simulink model "IntegratedStarterGenerator_lithium_ion"  (R2024b)
settings: Solver=ode23tb  StartTime=0.0  StopTime=15  FixedStep=1e-6  RelTol=1e-4  EnableMultiTasking=on
PreLoadFcn:
  | BeltStarterGeneratorData;
model workspace (MAT data in the model file):
  Cdc = 0.001
  ID_MAP = [-155.095933536 -155.095933536 -155.095933536 -155.095933536 -155.095933536 -155.095933536 -155.095933536 -155.095933536 -200.847752045 -245.560073478 -288.511134519 -330.698372533 ... (48076 elements, 28x101x17)]
  IQ_MAP = [-234.678365656 -234.678365656 -234.678365656 -234.678365656 -234.678365656 -234.678365656 -234.678365656 -234.678365656 -207.892729616 -187.030522468 -170.586354015 -157.025794022 ... (48076 elements, 28x101x17)]
  Ki_dcdc = 10
  Ki_id = 170
  Ki_iq = 170
  Ki_vdc = 100
  Kp_dcdc = 0.5
  Kp_id = 0.24
  Kp_iq = 0.24
  Kp_vdc = 20
  L0 = 5e-05
  Ld = 0.00011
  Lq = 0.00011
  Pmax = 140
  RPM_VECT = [0 1000 2000 3000 4000 5000 6000 7000 8000 9000 10000]
  R_f : Simulink.Parameter (value not decoded)
  Rs = 0.085
  TQ_VECT = [-3.5 -3.43 -3.36 -3.29 -3.22 -3.15 -3.08 -3.01 -2.94 -2.87 -2.8 -2.73 ... (101 elements, 1x101)]
  Tmax = 3.5
  Ts = 5e-06
  Tsi = 0.0001
  VDC_VECT = [8 8.625 9.25 9.875 10.5 11.125 11.75 12.375 13 13.625 14.25 14.875 ... (17 elements, 1x17)]
  dend_id = [1 -0.966796355036]
  dend_iq = [1 -0.900395111642]
  fsw = 5000
  fswd = 5000
  numd_id = 0.0332036449638
  numd_iq = 0.099604888358
  p = 3
  psim = 0.0159
  r_tire : Simulink.Parameter (value not decoded)
  tout = [0 5e-06 1e-05 1.5e-05 2e-05 2.5e-05 3e-05 3.5e-05 4e-05 4.5e-05 5e-05 5.5e-05 ... (200005 elements, 200005x1)]
symbols that are objects in the model workspace (value not decoded): R_f, r_tire
undefined symbols (not defined in the file or in its folder): DiscIntNeverNeededParam
libraries: fl_lib x51, nesl_utility x26, simulink x12, ee_lib x6, eeDiscretePi x3, sdl_lib x2, eeTransforms x2, batteryecm_lib x1, eePmsmCurrentController x1, eePmsmCurrentReferenceGen x1, eePmsmTorqueEstimator x1, eePwmGeneratorTwoLevel x1
(part 2 of 3)

== system IntegratedStarterGenerator_lithium_ion/Current sensor ==
  Current Sensor : fl_lib/Electrical/Electrical Sensors/Current Sensor
  PS-Simulink Converter1 : nesl_utility/PS-Simulink Converter  PhysicalDomain=network_engine_domain  SubClassName=ps_output  LeftPortType=input  RightPortType=output  PseudoPeriodic=off  Frequencies=[]  VectorFormat=1-D array  Unit=A  AffineConversion=off
  + : PMIOPort  Side=Left
  - : PMIOPort  Port=2  Side=Right
  tag scope: i_batt=global
  wires:
  PS-Simulink Converter1/1 -> [i_batt]
  connections:
  Current Sensor/RConn1 -- PS-Simulink Converter1/LConn1
  Current Sensor/LConn1 -- +/RConn1
  -/RConn1 -- Current Sensor/RConn2

== system IntegratedStarterGenerator_lithium_ion/Current sensor1 ==
  Current Sensor : fl_lib/Electrical/Electrical Sensors/Current Sensor
  PS-Simulink Converter1 : nesl_utility/PS-Simulink Converter  PhysicalDomain=network_engine_domain  SubClassName=ps_output  LeftPortType=input  RightPortType=output  PseudoPeriodic=off  Frequencies=[]  VectorFormat=1-D array  Unit=A  AffineConversion=off
  + : PMIOPort  Side=Left
  - : PMIOPort  Port=2  Side=Right
  tag scope: idc=global
  wires:
  PS-Simulink Converter1/1 -> [idc]
  connections:
  Current Sensor/RConn1 -- PS-Simulink Converter1/LConn1
  Current Sensor/LConn1 -- +/RConn1
  -/RConn1 -- Current Sensor/RConn2

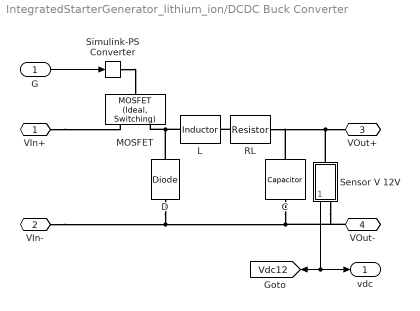
== system IntegratedStarterGenerator_lithium_ion/DCDC Buck Converter ==
  G : Inport
  C : fl_lib/Electrical/Electrical Elements/Capacitor  c=100 uF  r=1e-6 Ohm  g=0 1/Ohm  i_specify=off  i_priority=None  i=0 A  i_nominal_specify=off  i_nominal_value=1  i_nominal_unit=A  v_specify=off  v_priority=None  v=0 V  v_nominal_specify=off  v_nominal_value=1  v_nominal_unit=V  vc_specify=on  vc_priority=Low  vc=0 V  vc_nominal_specify=off  vc_nominal_value=1  vc_nominal_unit=V
  D : fl_lib/Electrical/Electrical Elements/Diode  Vf=0.6 V  Ron=0.3 Ohm  Goff=1e-8 1/Ohm  i_specify=off  i_priority=None  i=0 A  i_nominal_specify=off  i_nominal_value=1  i_nominal_unit=A  v_specify=off  v_priority=None  v=0 V  v_nominal_specify=off  v_nominal_value=1  v_nominal_unit=V
  L : fl_lib/Electrical/Electrical Elements/Inductor  l=3.7 mH  r=0 Ohm  g=1e-9 1/Ohm  i_specify=off  i_priority=None  i=0 A  i_nominal_specify=off  i_nominal_value=1  i_nominal_unit=A  v_specify=off  v_priority=None  v=0 V  v_nominal_specify=off  v_nominal_value=1  v_nominal_unit=V  i_L_specify=on  i_L_priority=Low  i_L=0 A  i_L_nominal_specify=off  i_L_nominal_value=1  i_L_nominal_unit=A
  MOSFET : ee_lib/Semiconductors & Converters/MOSFET (Ideal, Switching)  port_option=ee.enum.controlport.ps  Rds=0.01 Ohm  Goff=1e-6 1/Ohm  Vth=0.5 V  diode_param=2  diode_Vf=0.8 V  diode_Ron=0.001 Ohm  diode_Goff=1e-5 1/Ohm  diode_C=5e-8 F  diode_iRM=-235 A  diode_iF=300 A  diode_idot=-50 A/us  diode_trr_param=1  diode_trr_factor=3  diode_trr=15 us  diode_Qrr=1.5e+3 s*uA  ids_specify=off  ids_priority=None  ids=0 A  ids_nominal_specify=off  ids_nominal_value=1  ids_nominal_unit=A  vds_specify=off  vds_priority=None  vds=0 V  vds_nominal_specify=off  vds_nominal_value=1  vds_nominal_unit=V  vgs_specify=off  vgs_priority=None  vgs=0 V  vgs_nominal_specify=off  vgs_nominal_value=1  vgs_nominal_unit=V  thermal_loss_option=ee.enum.converters.thermalLossOption.constantvalues  Von_data=[0, 1.1, 1.3, 1.45, 1.75, 2.25, 2.7; 0, 1, 1.15, 1.35, 1.7, 2.35, 3] V  Tj=[298.15, 398.15] K  Iout_data=[0, 10, 50, 100, 200, 400, 600] A  Eon_data=[0, .29, 1.43, 2.86, 5.71, 13.14, 22.86; 0, .57, 2.63, 5.14, 10.29, 20.57, 30.29] * 1e-3 J  Eoff_data=[0, .21, 1.07, 2.14, 4.29, 9.86, 17.14; 0, .43, 1.97, 3.86, 7.71, 15.43, 22.71] * 1e-3 J  Eon_data_3D=[zeros(2, 5, 3)] J  Eoff_data_3D=[zeros(2, 5, 3)] J  Tj_loss=[298.15, 398.15] K  Iout_data_loss=[0, 10, 50, 100, 200, 400, 600] A  tabulateWithVds=false  Vds_loss=[0, 150, 300] V  Eon_scalar=22.86e-3 J  Eoff_scalar=17.14e-3 J  Voff=300 V  Iout_scalar=600 A  useCurrentFromPreviousCycle=false  useVoltageFromPreviousCycle=false  diodeModelType=ee.enum.converters.diodeModelType.pwl  diodeTableType=ee.enum.diode.tableType.IfMat  diode_ReverseIVType=ee.enum.diode.diodeReverseIV.constant  diode_IfMat=[.07, .12, .19, 1.75, 4.24, 7.32, 11.2; .16, .3, .72, 2.14, 4.02, 6.35, 9.12] A  diode_VfMat=[.9, 1.15, 1.25, 1.5, 1.75, 2.17, 2.6, 2.85; .58, .68, .75, 1.1, 1.38, 1.77, 2.27, 2.7] V  diode_TjVec=[25, 125] degC  diode_VfVec=[.5, .7, .9, 1.3, 1.7, 2.1, 2.5] V  diode_IfVec=[.1, .2, .5, 1, 2, 4, 7, 10] A  diode_IrMat=[1e-06, 2e-06, 5e-06, 1e-05, 2.5e-05, 5e-05, .0001; 2e-06, 5e-06, 1e-05, 4e-05, 8e-05, .0002, .0005] A  diode_VrMat=[10, 100, 200, 250, 300, 325, 350; 10, 70, 160, 220, 270, 300, 320] V  diode_VrVec=[10, 20, 40, 50, 70, 80, 100] V  diode_IrVec=[1e-06, 2e-06, 5e-06, 1e-05, 2e-05, 5e-05, .0001] A  diode_Vr=-600 V  diode_Ls=150 nH  diode_Erec=0.03 J  diode_rec_loss_model=ee.enum.diode.reverseRecoveryModel.fixed  diode_ErecVal=0 J  diode_scaleWithIandV=true  diode_ErecMat=zeros(2, 3) J  diode_TjrecVec=[298.15, 398.15] K  diode_IfrecVec=[.1, 1, 10] A  diode_IrecVal=10 A  diode_VrecVal=10 V  diode_tFilter=1 / 1000 / 100 s  separateThermalPortForDiode=false  thermal_network_parameterization=ee.enum.thermalNetworkTopology.external  Rth=[.03, .2] K/W  Rth_Cauer=[.03, .1, .2] K/W  Rth_Foster=[.03, .2] K/W  thermal_mass_parameterization=ee.enum.thermalNetwork.timeconstant  thermal_mass=[3, 25] J/K  thermal_mass_Cauer=[3, 10, 25] J/K  thermal_mass_Foster=[33, 50] J/K  thermal_time_constant=[.1, 5] s  thermal_time_constant_Cauer=[.1, 1, 5] s  thermal_time_constant_Foster=[1, 10] s  thermal_mass_initial_temperatures=[25, 25] degC  thermal_mass_initial_temperatures_Cauer=[25, 25, 25] degC  junction_thermal_mass=0.1 J/K  Tvec_initial_Foster=[25, 25, 25, 25] degC  RthDiode=[.03, .2] K/W  RthCauerDiode=[.03, .1, .2] K/W  RthFosterDiode=[.03, .2] K/W  thermalMassDiode=[3, 25] J/K  thermalMassCauerDiode=[3, 10, 25] J/K  thermalMassFosterDiode=[33, 50] J/K  thermalTauDiode=[.1, 5] s  thermalTauCauerDiode=[.1, 1, 5] s  thermalTauFosterDiode=[1, 10] s  thermalMassInitTempDiode=[25, 25] degC  thermalMassInitTempCauerDiode=[25, 25, 25] degC  junctionthermalMassDiode=0.1 J/K  TVecInitialFosterDiode=[25, 25, 25, 25] degC  no_thermal_network=0  mosfet_junction_temperature_specify=off  mosfet_junction_temperature_priority=None  mosfet_junction_temperature=25 degC  mosfet_junction_temperature_nominal_specify=off  mosfet_junction_temperature_nominal_value=1  mosfet_junction_temperature_nominal_unit=degC  diode_junction_temperature_specify=off  diode_junction_temperature_priority=None  diode_junction_temperature=25 degC  diode_junction_temperature_nominal_specify=off  diode_junction_temperature_nominal_value=1  diode_junction_temperature_nominal_unit=degC  Qj_specify=off  Qj_priority=None  Qj=0 W  Qj_nominal_specify=off  Qj_nominal_value=1  Qj_nominal_unit=W  accumulatedSwitchingLosses_specify=off  accumulatedSwitchingLosses_priority=None  accumulatedSwitchingLosses=0 J
  RL : fl_lib/Electrical/Electrical Elements/Resistor  R=1.5 Ohm  i_specify=off  i_priority=None  i=0 A  i_nominal_specify=off  i_nominal_value=1  i_nominal_unit=A  v_specify=off  v_priority=None  v=0 V  v_nominal_specify=off  v_nominal_value=1  v_nominal_unit=V
  Sensor V 12V : Subsystem
  Simulink-PS Converter : nesl_utility/Simulink-PS Converter  PhysicalDomain=network_engine_domain  SubClassName=ps_input  LeftPortType=input  RightPortType=output  PseudoPeriodic=off  Frequencies=[]  NoiseDistribution=none  NoiseParameters=[]  Unit=1  AffineConversion=off  FilteringAndDerivatives=zero  SimscapeFilterOrder=1  InputFilterTimeConstant=0.001  UdotUserProvided=1
  VIn+ : PMIOPort  Side=Left
  VIn- : PMIOPort  Port=2  Side=Left
  VOut+ : PMIOPort  Port=3  Side=Right
  VOut- : PMIOPort  Port=4  Side=Right
  vdc : Outport  VectorParamsAs1DForOutWhenUnconnected=off
  tag scope: Vdc12=global
  wires:
  G/1 -> Simulink-PS Converter/1
  Sensor V 12V/1(vdc) -> [Vdc12], vdc/1
  connections:
  VIn-/RConn1 -- D/LConn1 -- Sensor V 12V/RConn1 -- VOut-/RConn1 -- C/RConn1
  Simulink-PS Converter/RConn1 -- MOSFET/LConn1
  L/LConn1 -- D/RConn1 -- MOSFET/RConn2
  VIn+/RConn1 -- MOSFET/RConn1
  RL/LConn1 -- L/RConn1
  C/LConn1 -- RL/RConn1 -- VOut+/RConn1 -- Sensor V 12V/LConn1

== system IntegratedStarterGenerator_lithium_ion/DCDC Controller ==
  Ref : Inport
  Vdc : Inport  Port=2
  Constant : Constant  Value=0  SampleTime=-1
  Discrete PI Controller with Integral Anti-Windup : eeDiscretePi/Discrete PI Controller with Integral Anti-Windup  Kp=Kp_dcdc  Ki=Ki_dcdc  x0=0  B=1  A=0  Ts=1e-3
  PWM Generation : Subsystem  mask{f=fswd, Ts=Ts}
      mask prompts: f "Switching frequency"; Ts "Sample time"
  Rate Transition : RateTransition  OutPortSampleTime=1e-3
  Rate Transition2 : RateTransition
  Sum : Sum  Inputs=|+-
  G : Outport  VectorParamsAs1DForOutWhenUnconnected=off
  wires:
  Vdc/1 -> Rate Transition/1
  Rate Transition2/1 -> PWM Generation/1(DC)
  Ref/1 -> Sum/1
  Rate Transition/1 -> Sum/2
  PWM Generation/1(PWM) -> G/1
  Sum/1 -> Discrete PI Controller with Integral Anti-Windup/1
  Discrete PI Controller with Integral Anti-Windup/1 -> Rate Transition2/1
  Constant/1 -> Discrete PI Controller with Integral Anti-Windup/2

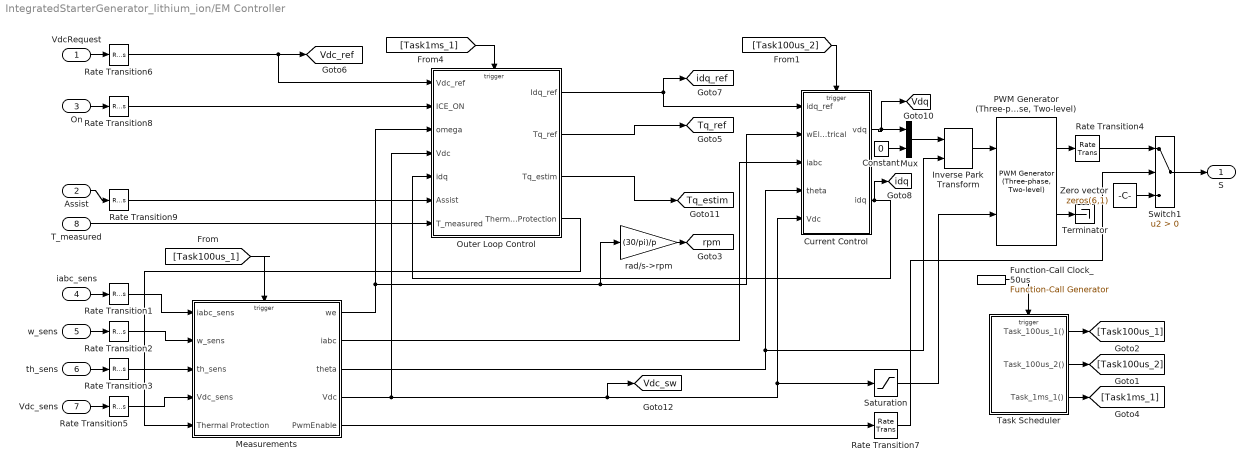
== system IntegratedStarterGenerator_lithium_ion/EM Controller ==
  VdcRequest : Inport
  Assist : Inport  Port=2
  On : Inport  Port=3
  iabc_sens : Inport  Port=4
  w_sens : Inport  Port=5
  th_sens : Inport  Port=6
  Vdc_sens : Inport  Port=7
  T_measured : Inport  Port=8
  Constant : Constant  Value=0  SampleTime=-1
  Current Control : Subsystem
  Function-Call Clock_50us : simulink/Ports & Subsystems/Function-Call Generator  sample_time=5e-5  numberOfIterations=1  DisallowWideOutput=off
  Inverse Park Transform : eeTransforms/Inverse Park Transform  AxisAlignment=Q-axis  PowerInvariant=off
  Measurements : Subsystem
  Mux : Mux  Inputs=2
  Outer Loop Control : Subsystem
  "PWM Generator (Three-phase, Two-level)" : eePwmGeneratorTwoLevel/PWM Generator (Three-phase, Two-level)  PWMMode=Continuous PWM (CPWM)  CPWMMode=SPWM: sinusoidal PWM  DPWMMode=60 DPWM: 60 degree discontinuous PWM  fsw=fsw  Ts=Ts
  Rate Transition{1..9} (9 alike) : RateTransition
  Saturation : Saturate  UpperLimit=500  LowerLimit=10
  Switch1 : Switch  Criteria=u2 > Threshold  SaturateOnIntegerOverflow=off  InputSameDT=off
  Task Scheduler : Stateflow chart  TreatAsAtomicUnit=on
  Terminator : Terminator
  Zero vector : Constant  Value=zeros(6,1)
  rad/s->rpm : Gain  Gain=(30/pi)/p
  S : Outport  VectorParamsAs1DForOutWhenUnconnected=off
  tag scope: Tq_estim=global, Tq_ref=global, Vdc_ref=global, Vdc_sw=global, Vdq=global, idq=global, idq_ref=global, rpm=global
  wires:
  Measurements/4(Vdc) -> Current Control/5(Vdc), Saturation/1, [Vdc_sw], Outer Loop Control/4(Vdc)
  [Task1ms_1] -> Outer Loop Control/Trigger
  Rate Transition8/1 -> Outer Loop Control/2(ICE_ON)
  Rate Transition1/1 -> Measurements/1(iabc_sens)
  Switch1/1 -> S/1
  Rate Transition5/1 -> Measurements/4(Vdc_sens)
  Current Control/1(vdq) -> [Vdq], Mux/1
  Current Control/2(idq) -> [idq], Outer Loop Control/5(idq)
  Outer Loop Control/1(Idq_ref) -> [idq_ref], Current Control/1(idq_ref)
  Task Scheduler/1(Task_100us_1()) -> [Task100us_1]
  Measurements/3(theta) -> Current Control/4(theta), Inverse Park Transform/2
  Rate Transition4/1 -> Switch1/1
  Outer Loop Control/3(Tq_estim) -> [Tq_estim]
  Rate Transition7/1 -> Switch1/2
  VdcRequest/1 -> Rate Transition6/1
  Zero vector/1 -> Switch1/3
  Measurements/1(we) -> Outer Loop Control/3(omega), Current Control/2(wElectrical), rad/s->rpm/1
  th_sens/1 -> Rate Transition3/1
  On/1 -> Rate Transition8/1
  Outer Loop Control/2(Tq_ref) -> [Tq_ref]
  Rate Transition6/1 -> [Vdc_ref], Outer Loop Control/1(Vdc_ref)
  iabc_sens/1 -> Rate Transition1/1
  Task Scheduler/3(Task_1ms_1()) -> [Task1ms_1]
  Rate Transition3/1 -> Measurements/3(th_sens)
  Function-Call Clock_50us/1 -> Task Scheduler/Trigger
  Measurements/5(PwmEnable) -> Rate Transition7/1
  "PWM Generator (Three-phase, Two-level)"/2 -> Terminator/1
  Rate Transition2/1 -> Measurements/2(w_sens)
  Saturation/1 -> "PWM Generator (Three-phase, Two-level)"/2
  [Task100us_2] -> Current Control/Trigger
  w_sens/1 -> Rate Transition2/1
  rad/s->rpm/1 -> [rpm]
  Inverse Park Transform/1 -> "PWM Generator (Three-phase, Two-level)"/1
  "PWM Generator (Three-phase, Two-level)"/1 -> Rate Transition4/1
  Vdc_sens/1 -> Rate Transition5/1
  Task Scheduler/2(Task_100us_2()) -> [Task100us_2]
  [Task100us_1] -> Measurements/Trigger
  Measurements/2(iabc) -> Current Control/3(iabc)
  Mux/1 -> Inverse Park Transform/1
  Constant/1 -> Mux/2
  Assist/1 -> Rate Transition9/1
  Rate Transition9/1 -> Outer Loop Control/6(Assist)
  T_measured/1 -> Outer Loop Control/7(T_measured)
  Outer Loop Control/4(Thermal Protection) -> Measurements/5(Thermal Protection)

== system IntegratedStarterGenerator_lithium_ion/Gate Driver ==
  S : Inport
  Demux : Demux  Outputs=6
  Simulink-PS Converter{1..6} (6 alike) : nesl_utility/Simulink-PS Converter  PhysicalDomain=network_engine_domain  SubClassName=ps_input  LeftPortType=input  RightPortType=output  PseudoPeriodic=off  Frequencies=[]  NoiseDistribution=none  NoiseParameters=[]  Unit=1  AffineConversion=off  FilteringAndDerivatives=zero  SimscapeFilterOrder=1  InputFilterTimeConstant=0.001  UdotUserProvided=1
  Six-Pulse Gate Multiplexer : ee_lib/Semiconductors & Converters/Converters/Six-Pulse Gate Multiplexer  port_option=ee.enum.controlport.ps
  G : PMIOPort  Side=Right
  wires:
  Demux/1 -> Simulink-PS Converter1/1
  S/1 -> Demux/1
  Demux/4 -> Simulink-PS Converter4/1
  Demux/2 -> Simulink-PS Converter2/1
  Demux/3 -> Simulink-PS Converter3/1
  Demux/5 -> Simulink-PS Converter5/1
  Demux/6 -> Simulink-PS Converter6/1
  connections:
  Six-Pulse Gate Multiplexer/RConn1 -- G/RConn1
  Simulink-PS Converter1/RConn1 -- Six-Pulse Gate Multiplexer/LConn1
  Simulink-PS Converter3/RConn1 -- Six-Pulse Gate Multiplexer/LConn3
  Simulink-PS Converter5/RConn1 -- Six-Pulse Gate Multiplexer/LConn5
  Simulink-PS Converter6/RConn1 -- Six-Pulse Gate Multiplexer/LConn6
  Simulink-PS Converter4/RConn1 -- Six-Pulse Gate Multiplexer/LConn4
  Simulink-PS Converter2/RConn1 -- Six-Pulse Gate Multiplexer/LConn2

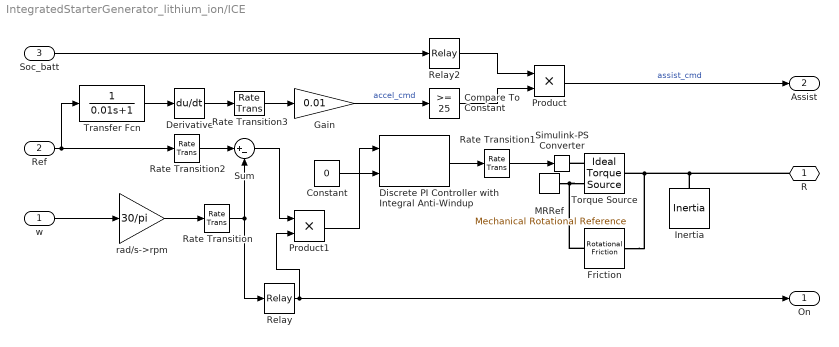
== system IntegratedStarterGenerator_lithium_ion/ICE ==
  w : Inport
  Ref : Inport  Port=2
  Soc_batt : Inport  Port=3
  Compare To Constant : simulink/Logic and Bit Operations/Compare To Constant  relop=>=  const=25  OutDataTypeStr=boolean
  Constant : Constant  Value=0  SampleTime=0.01
  Derivative : Derivative  CoefficientInTFapproximation=0.05
  Discrete PI Controller with Integral Anti-Windup : eeDiscretePi/Discrete PI Controller with Integral Anti-Windup  Kp=0.5  Ki=0.4  x0=0  B=6.5  A=-0.1*Tmax  Ts=0.0001
  Friction : fl_lib/Mechanical/Rotational Elements/Rotational Friction  brkwy_trq=0.01e-3 N*m  brkwy_vel=0.05 rad/s  Col_trq=0.01e-3 N*m  visc_coef=0.0005 N*m/(rad/s)  w_specify=off  w_priority=None  w=0 rad/s  w_nominal_specify=off  w_nominal_value=1  w_nominal_unit=rad/s  t_specify=off  t_priority=None  t=0 N*m  t_nominal_specify=off  t_nominal_value=1  t_nominal_unit=N*m
  Gain : Gain  Gain=0.01
  Inertia : fl_lib/Mechanical/Rotational Elements/Inertia  inertia=0.0025 kg*m^2  num_ports=foundation.enum.numPorts2.one  w_specify=on  w_priority=Low  w=0 rad/s  w_nominal_specify=off  w_nominal_value=1  w_nominal_unit=rad/s  t_specify=off  t_priority=None  t=0 N*m  t_nominal_specify=off  t_nominal_value=1  t_nominal_unit=N*m
  MRRef : fl_lib/Mechanical/Rotational Elements/Mechanical Rotational Reference
  Product : Product
  Product1 : Product
  Rate Transition : RateTransition  OutPortSampleTime=0.0001
  Rate Transition1 : RateTransition
  Rate Transition2 : RateTransition  OutPortSampleTime=0.0001
  Rate Transition3 : RateTransition  OutPortSampleTime=0.0001
  Relay : Relay  OnSwitchValue=950  OffSwitchValue=850  ZeroCross=off
  Relay2 : Relay  OnSwitchValue=0.5  OffSwitchValue=0.2  ZeroCross=off
  Simulink-PS Converter : nesl_utility/Simulink-PS Converter  PhysicalDomain=network_engine_domain  SubClassName=ps_input  LeftPortType=input  RightPortType=output  PseudoPeriodic=off  Frequencies=[]  NoiseDistribution=none  NoiseParameters=[]  Unit=N*m  AffineConversion=off  FilteringAndDerivatives=zero  SimscapeFilterOrder=1  InputFilterTimeConstant=0.001  UdotUserProvided=1
  Sum : Sum  Inputs=|+-
  Torque Source : fl_lib/Mechanical/Mechanical Sources/Ideal Torque Source
  Transfer Fcn : TransferFcn  Denominator=[0.01 1]
  rad/s->rpm : Gain  Gain=30/pi
  R : PMIOPort  Side=Right
  On : Outport  VectorParamsAs1DForOutWhenUnconnected=off
  Assist : Outport  Port=2
  wires:
  Rate Transition1/1 -> Simulink-PS Converter/1
  rad/s->rpm/1 -> Rate Transition/1
  Relay/1 -> Product1/2, On/1
  w/1 -> rad/s->rpm/1
  Ref/1 -> Transfer Fcn/1, Rate Transition2/1
  Rate Transition/1 -> Relay/1, Sum/2
  Sum/1 -> Product1/1
  Discrete PI Controller with Integral Anti-Windup/1 -> Rate Transition1/1
  Constant/1 -> Discrete PI Controller with Integral Anti-Windup/2
  Rate Transition2/1 -> Sum/1
  Gain/1 -> Compare To Constant/1  "accel_cmd"
  Transfer Fcn/1 -> Derivative/1
  Derivative/1 -> Rate Transition3/1
  Soc_batt/1 -> Relay2/1
  Relay2/1 -> Product/1
  Compare To Constant/1 -> Product/2
  Product/1 -> Assist/1  "assist_cmd"
  Rate Transition3/1 -> Gain/1
  Product1/1 -> Discrete PI Controller with Integral Anti-Windup/1
  connections:
  R/RConn1 -- Inertia/LConn1 -- Torque Source/LConn1 -- Friction/LConn1
  MRRef/LConn1 -- Friction/RConn1 -- Torque Source/RConn2
  Torque Source/RConn1 -- Simulink-PS Converter/RConn1

== system IntegratedStarterGenerator_lithium_ion/Low-Batt_cutoff ==
  S : Inport
  Rate Transition : RateTransition
  Relay2 : Relay  OnSwitchValue=0.75  OffSwitchValue=0.6  ZeroCross=off
  SPST Switch : ee_lib/Switches & Breakers/SPST Switch  R_closed=0.01 Ohm  G_open=1e-6 S  Threshold=0.5 V  Width=0 V  model_dynamics=0  t_on=1e-3 s  t_off=1e-3 s  initial_vT=0 V
      settings: InternalSimscapePortConfiguration="{\"Bottom\":[],\"Left\":[{\"id\":\"vT\",\"label\":\"vT\",\"type\":\"input\"},{\"id\":\"p\",\"label\":\"\",\"type\":\"foundation.electrical.electrical\"}],\"Right\":[{\"id\":\"n\",\"label\":\"\",\"type\":\"foundation.electrical.electrical\"}],\"Top\":[]}"
  Simulink-PS Converter2 : nesl_utility/Simulink-PS Converter  PhysicalDomain=network_engine_domain  SubClassName=ps_input  LeftPortType=input  RightPortType=output  PseudoPeriodic=off  Frequencies=[]  NoiseDistribution=none  NoiseParameters=[]  Unit=1  AffineConversion=off  FilteringAndDerivatives=zero  SimscapeFilterOrder=1  InputFilterTimeConstant=0.001  UdotUserProvided=1
  a : PMIOPort  Side=Left
  b : PMIOPort  Port=2  Side=Right
  wires:
  Rate Transition/1 -> Simulink-PS Converter2/1
  S/1 -> Relay2/1
  Relay2/1 -> Rate Transition/1
  connections:
  SPST Switch/LConn2 -- a/RConn1
  SPST Switch/LConn1 -- Simulink-PS Converter2/RConn1
  SPST Switch/RConn1 -- b/RConn1

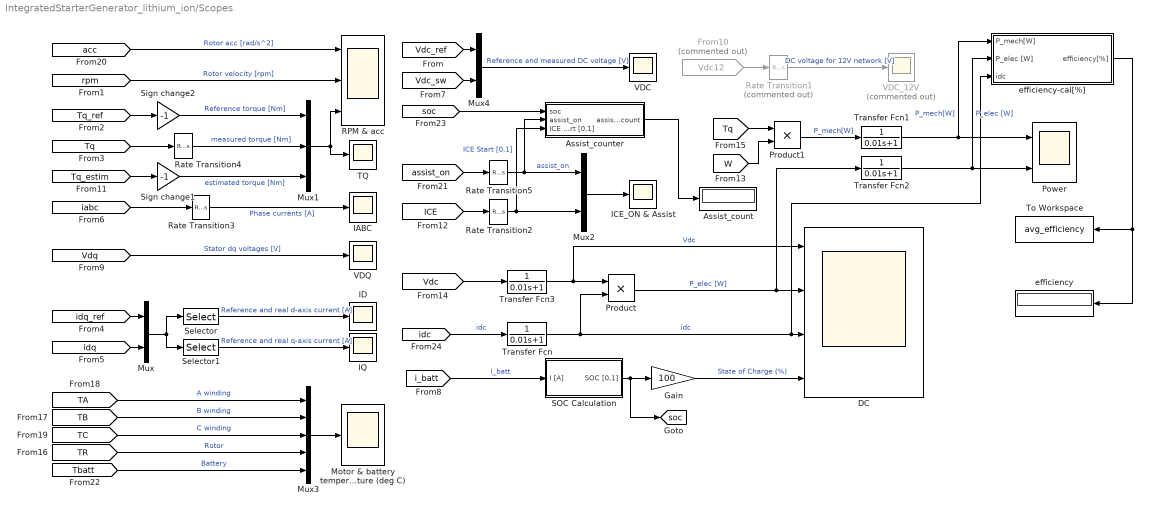
== system IntegratedStarterGenerator_lithium_ion/Scopes ==
  Assist_count : Display
  Assist_counter : Subsystem
  DC : Scope  NumInputPorts=4
  From10 : From  Commented=on  GotoTag=Vdc12  TagVisibility=global
  Gain : Gain  Gain=100
  IABC : Scope
  ICE_ON & Assist : Scope
  ID : Scope
  IQ : Scope
  Motor & battery temperature (deg C) : Scope
  Mux : Mux  Inputs=2
  Mux1 : Mux  Inputs=3
  Mux2 : Mux  Inputs=2
  Mux3 : Mux  Inputs=5
  Mux4 : Mux  Inputs=2
  Power : Scope  NumInputPorts=2
  Product : Product
  Product1 : Product
  RPM & acc : Scope  NumInputPorts=3
  Rate Transition1 : RateTransition  Commented=on  OutPortSampleTime=1e-4
  Rate Transition2 : RateTransition  OutPortSampleTime=1e-4
  Rate Transition3 : RateTransition  OutPortSampleTime=1e-4
  Rate Transition4 : RateTransition
  Rate Transition5 : RateTransition  OutPortSampleTime=1e-4
  SOC Calculation : Subsystem
  Selector : Selector  InputPortWidth=4  IndexOptions=Index vector (dialog)  Indices=[1 3]  OutputSizes=1
  Selector1 : Selector  InputPortWidth=4  IndexOptions=Index vector (dialog)  Indices=[2 4]  OutputSizes=1
  Sign change1 : Gain  Gain=-1
  Sign change2 : Gain  Gain=-1
  TQ : Scope
  To Workspace : ToWorkspace  VariableName=avg_efficiency  SaveFormat=Timeseries  SampleTime=-1
  Transfer Fcn{,1..3} (4 alike) : TransferFcn  Denominator=[0.01 1]
  VDC : Scope
  VDC_12V : Scope  Commented=on
  VDQ : Scope
  efficiency : Display
  efficiency-cal[%] : Subsystem
  tag scope: soc=global
  wires:
  [rpm] -> RPM & acc/2  "Rotor velocity [rpm]"
  Mux1/1 -> RPM & acc/3, TQ/1
  Selector/1 -> ID/1  "Reference and real d-axis current [A]"
  Selector1/1 -> IQ/1  "Reference and real q-axis current [A]"
  [iabc] -> Rate Transition3/1
  [Vdq] -> VDQ/1  "Stator dq voltages [V]"
  Mux4/1 -> VDC/1  "Reference and measured DC voltage [V]"
  [idq_ref] -> Mux/1
  [idq] -> Mux/2
  Mux/1 -> Selector1/1, Selector/1
  [Tq_estim] -> Sign change1/1
  [Vdc_sw] -> Mux4/2
  [Vdc_ref] -> Mux4/1
  Rate Transition3/1 -> IABC/1  "Phase currents [A]"
  From10/1 -> Rate Transition1/1
  Rate Transition1/1 -> VDC_12V/1  "DC voltage for 12V network [V]"
  [ICE] -> Rate Transition2/1
  [Tq_ref] -> Sign change2/1
  [Tq] -> Rate Transition4/1
  Sign change1/1 -> Mux1/3  "estimated torque [Nm]"
  Sign change2/1 -> Mux1/1  "Reference torque [Nm]"
  Product/1 -> Transfer Fcn2/1, DC/2  "P_elec [W]"
  SOC Calculation/1(SOC [0,1]) -> [soc], Gain/1
  [idc] -> Transfer Fcn/1  "idc"
  [Vdc] -> Transfer Fcn3/1
  Rate Transition4/1 -> Mux1/2  "measured torque [Nm]"
  [Tq] -> Product1/1
  [W] -> Product1/2
  Product1/1 -> Transfer Fcn1/1  "P_mech[W]"
  [TR] -> Mux3/4  "Rotor"
  [TC] -> Mux3/3  "C winding"
  [TB] -> Mux3/2  "B winding"
  Mux3/1 -> Motor & battery temperature (deg C)/1
  [TA] -> Mux3/1  "A winding"
  [acc] -> RPM & acc/1  "Rotor acc [rad/s^2]"
  Mux2/1 -> ICE_ON & Assist/1
  Rate Transition2/1 -> Mux2/2, Assist_counter/3(ICE Start [0,1])  "ICE Start [0,1]"
  [assist_on] -> Rate Transition5/1
  Rate Transition5/1 -> Assist_counter/2(assist_on), Mux2/1  "assist_on"
  Gain/1 -> DC/4  "State of Charge (%)"
  [Tbatt] -> Mux3/5  "Battery"
  [soc] -> Assist_counter/1(soc)
  Assist_counter/1(assist_count) -> Assist_count/1
  Transfer Fcn/1 -> Product/2, efficiency-cal[%]/3(idc), DC/3  "idc"
  Transfer Fcn1/1 -> efficiency-cal[%]/1(P_mech[W]), Power/1  "P_mech[W]"
  Transfer Fcn2/1 -> efficiency-cal[%]/2(P_elec [W]), Power/2  "P_elec [W]"
  Transfer Fcn3/1 -> DC/1, Product/1  "Vdc"
  [i_batt] -> SOC Calculation/1(I [A])  "I_batt"
  efficiency-cal[%]/1(efficiency[%]) -> efficiency/1, To Workspace/1

== system IntegratedStarterGenerator_lithium_ion/Sensing Temperature ==
  PS-Simulink Converter : nesl_utility/PS-Simulink Converter  PhysicalDomain=network_engine_domain  SubClassName=ps_output  LeftPortType=input  RightPortType=output  PseudoPeriodic=off  Frequencies=[]  VectorFormat=1-D array  Unit=degC  AffineConversion=on
  Temperature Sensor : fl_lib/Thermal/Thermal Sensors/Temperature Sensor  temperature_measure=foundation.enum.MeasurementReference.difference
  ThRef : fl_lib/Thermal/Thermal Elements/Thermal Reference
  H : PMIOPort  Side=Left
  tag scope: Tbatt=global
  wires:
  PS-Simulink Converter/1 -> [Tbatt]
  connections:
  Temperature Sensor/RConn2 -- PS-Simulink Converter/LConn1
  ThRef/LConn1 -- Temperature Sensor/RConn1
  H/RConn1 -- Temperature Sensor/LConn1

== system IntegratedStarterGenerator_lithium_ion/Sensor ICE Torque ==
  PS-Simulink Converter3 : nesl_utility/PS-Simulink Converter  PhysicalDomain=network_engine_domain  SubClassName=ps_output  LeftPortType=input  RightPortType=output  PseudoPeriodic=off  Frequencies=[]  VectorFormat=1-D array  Unit=N*m  AffineConversion=off
  Torque Sensor : fl_lib/Mechanical/Mechanical Sensors/Ideal Torque Sensor
  R : PMIOPort  Side=Left
  C : PMIOPort  Port=2  Side=Right
  tag scope: Tq=global
  wires:
  PS-Simulink Converter3/1 -> [Tq]
  connections:
  Torque Sensor/RConn2 -- PS-Simulink Converter3/LConn1
  Torque Sensor/RConn1 -- R/RConn1
  Torque Sensor/LConn1 -- C/RConn1

== system IntegratedStarterGenerator_lithium_ion/Sensor ICE Shaft ==
  MRRef : fl_lib/Mechanical/Rotational Elements/Mechanical Rotational Reference
  Motion Sensor : fl_lib/Mechanical/Mechanical Sensors/Ideal Rotational Motion Sensor  reference=foundation.enum.MeasurementReference.difference  acceleration_port=true  velocity_port=true  position_port=true  wrap_angle=simscape.enum.onoff.off  offset=0 deg
      settings: InternalSimscapePortConfiguration="{\"Bottom\":[],\"Left\":[{\"id\":\"R\",\"label\":\"R\",\"type\":\"foundation.mechanical.rotational.rotational\"}],\"Right\":[{\"id\":\"C\",\"label\":\"C\",\"type\":\"foundation.mechanical.rotational.rotational\"},{\"id\":\"alpha\",\"label\":\"α\",\"type\":\"output\"},{\"id\":\"W\",\"label\":\"W\",\"type\":\"output\"},{\"id\":\"A\",\"label\":\"A\",\"type\":\"output\"}],\"Top\":[]}"
  PS-Simulink Converter : nesl_utility/PS-Simulink Converter  PhysicalDomain=network_engine_domain  SubClassName=ps_output  LeftPortType=input  RightPortType=output  PseudoPeriodic=off  Frequencies=[]  VectorFormat=1-D array  Unit=rad  AffineConversion=off
  PS-Simulink Converter1 : nesl_utility/PS-Simulink Converter  PhysicalDomain=network_engine_domain  SubClassName=ps_output  LeftPortType=input  RightPortType=output  PseudoPeriodic=off  Frequencies=[]  VectorFormat=1-D array  Unit=rad/s^2  AffineConversion=off
  PS-Simulink Converter2 : nesl_utility/PS-Simulink Converter  PhysicalDomain=network_engine_domain  SubClassName=ps_output  LeftPortType=input  RightPortType=output  PseudoPeriodic=off  Frequencies=[]  VectorFormat=1-D array  Unit=rad/s  AffineConversion=off
  R : PMIOPort  Side=Left
  W : Outport  VectorParamsAs1DForOutWhenUnconnected=off
  A : Outport  Port=2  VectorParamsAs1DForOutWhenUnconnected=off
  acc : Outport  Port=3
  wires:
  PS-Simulink Converter/1 -> A/1
  PS-Simulink Converter2/1 -> W/1
  PS-Simulink Converter1/1 -> acc/1
  connections:
  Motion Sensor/RConn3 -- PS-Simulink Converter2/LConn1
  MRRef/LConn1 -- Motion Sensor/RConn1
  Motion Sensor/RConn2 -- PS-Simulink Converter1/LConn1
  Motion Sensor/LConn1 -- R/RConn1
  Motion Sensor/RConn4 -- PS-Simulink Converter/LConn1

== system IntegratedStarterGenerator_lithium_ion/Sensor Phase Currents ==
  Current Sensor : ee_lib/Sensors & Transducers/Current Sensor (Three-Phase)
  PS-Simulink Converter : nesl_utility/PS-Simulink Converter  PhysicalDomain=network_engine_domain  SubClassName=ps_output  LeftPortType=input  RightPortType=output  PseudoPeriodic=off  Frequencies=[]  VectorFormat=1-D array  Unit=A  AffineConversion=off
  1 : PMIOPort  Side=Left
  2 : PMIOPort  Port=2  Side=Right
  tag scope: iabc=global
  wires:
  PS-Simulink Converter/1 -> [iabc]
  connections:
  1/RConn1 -- Current Sensor/LConn1
  Current Sensor/RConn1 -- PS-Simulink Converter/LConn1
  2/RConn1 -- Current Sensor/RConn2

== system IntegratedStarterGenerator_lithium_ion/Switch 12V Load ==
  S : Inport
  Simulink-PS Converter2 : nesl_utility/Simulink-PS Converter  PhysicalDomain=network_engine_domain  SubClassName=ps_input  LeftPortType=input  RightPortType=output  PseudoPeriodic=off  Frequencies=[]  NoiseDistribution=none  NoiseParameters=[]  Unit=1  AffineConversion=off  FilteringAndDerivatives=zero  SimscapeFilterOrder=1  InputFilterTimeConstant=0.001  UdotUserProvided=1
  Switch : fl_lib/Electrical/Electrical Elements/Switch  R_closed=0.01 Ohm  G_open=1e-8 1/Ohm  Threshold=0  i_specify=off  i_priority=None  i=0 A  i_nominal_specify=off  i_nominal_value=1  i_nominal_unit=A  v_specify=off  v_priority=None  v=0 V  v_nominal_specify=off  v_nominal_value=1  v_nominal_unit=V
  a : PMIOPort  Side=Left
  b : PMIOPort  Port=2  Side=Right
  wires:
  S/1 -> Simulink-PS Converter2/1
  connections:
  b/RConn1 -- Switch/LConn1
  Simulink-PS Converter2/RConn1 -- Switch/RConn1
  Switch/RConn2 -- a/RConn1

== system IntegratedStarterGenerator_lithium_ion/Switch Load ==
  S : Inport
  Rate Transition : RateTransition
  Simulink-PS Converter2 : nesl_utility/Simulink-PS Converter  PhysicalDomain=network_engine_domain  SubClassName=ps_input  LeftPortType=input  RightPortType=output  PseudoPeriodic=off  Frequencies=[]  NoiseDistribution=none  NoiseParameters=[]  Unit=1  AffineConversion=on  FilteringAndDerivatives=zero  SimscapeFilterOrder=1  InputFilterTimeConstant=0.001  UdotUserProvided=1
  Switch : fl_lib/Electrical/Electrical Elements/Switch  R_closed=0.01 Ohm  G_open=1e-8 1/Ohm  Threshold=0  i_specify=off  i_priority=None  i=0 A  i_nominal_specify=off  i_nominal_value=1  i_nominal_unit=A  v_specify=off  v_priority=None  v=0 V  v_nominal_specify=off  v_nominal_value=1  v_nominal_unit=V
  a : PMIOPort  Side=Left
  b : PMIOPort  Port=2  Side=Right
  wires:
  S/1 -> Rate Transition/1
  Rate Transition/1 -> Simulink-PS Converter2/1
  connections:
  Switch/RConn2 -- a/RConn1
  Simulink-PS Converter2/RConn1 -- Switch/RConn1
  b/RConn1 -- Switch/LConn1

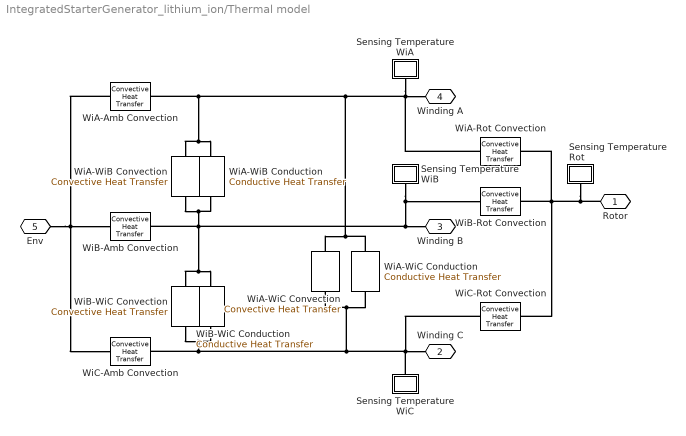
== system IntegratedStarterGenerator_lithium_ion/Thermal model ==
  Sensing Temperature Rot : Subsystem
      mask Display: disp('TR')
  Sensing Temperature WiA : Subsystem
      mask Display: disp('TA')
  Sensing Temperature WiB : Subsystem
      mask Display: disp('TB')
  Sensing Temperature WiC : Subsystem
      mask Display: disp('TC')
  WiA-Amb Convection : fl_lib/Thermal/Thermal Elements/Convective Heat Transfer  thermal_type=foundation.enum.constant_variable.constant  area=0.1 m^2  heat_tr_coeff=0.2 W/(m^2 * K)  min_heat_tr_coeff=1e-3 W/(K*m^2)  T_specify=off  T_priority=None  T=0 K  T_nominal_specify=off  T_nominal_value=1  T_nominal_unit=K  Q_specify=off  Q_priority=None  Q=0 J/s  Q_nominal_specify=off  Q_nominal_value=1  Q_nominal_unit=J/s
  WiA-Rot Convection : fl_lib/Thermal/Thermal Elements/Convective Heat Transfer  thermal_type=foundation.enum.constant_variable.constant  area=0.02 m^2  heat_tr_coeff=2 W/(m^2 * K)  min_heat_tr_coeff=1e-3 W/(K*m^2)  T_specify=off  T_priority=None  T=0 K  T_nominal_specify=off  T_nominal_value=1  T_nominal_unit=K  Q_specify=off  Q_priority=None  Q=0 J/s  Q_nominal_specify=off  Q_nominal_value=1  Q_nominal_unit=J/s
  WiA-WiB Conduction : fl_lib/Thermal/Thermal Elements/Conductive Heat Transfer  thermal_type=foundation.enum.ConstantVariableTabulated.Constant  wall_geometry=foundation.enum.ConductionWallGeometry.Planar  area=0.002 m^2  thickness=0.1 m  d_in=0.05 m  d_out=0.1 m  L=1 m  th_cond_min=10 W/(K*m)  th_cond=0.8 W/(m*K)  th_cond_TLU=[413, 401, 392, 383, 371, 357, 342] W/(K*m)  temp_TLU=[200, 273, 400, 600, 800, 1000, 1200] K  T_specify=off  T_priority=None  T=0 K  T_nominal_specify=off  T_nominal_value=1  T_nominal_unit=K  Q_specify=off  Q_priority=None  Q=0 J/s  Q_nominal_specify=off  Q_nominal_value=1  Q_nominal_unit=J/s
  WiA-WiB Convection : fl_lib/Thermal/Thermal Elements/Convective Heat Transfer  thermal_type=foundation.enum.constant_variable.constant  area=0.004 m^2  heat_tr_coeff=2 W/(m^2 * K)  min_heat_tr_coeff=1e-3 W/(K*m^2)  T_specify=off  T_priority=None  T=0 K  T_nominal_specify=off  T_nominal_value=1  T_nominal_unit=K  Q_specify=off  Q_priority=None  Q=0 J/s  Q_nominal_specify=off  Q_nominal_value=1  Q_nominal_unit=J/s
  WiA-WiC Conduction : fl_lib/Thermal/Thermal Elements/Conductive Heat Transfer  thermal_type=foundation.enum.ConstantVariableTabulated.Constant  wall_geometry=foundation.enum.ConductionWallGeometry.Planar  area=0.002 m^2  thickness=0.1 m  d_in=0.05 m  d_out=0.1 m  L=1 m  th_cond_min=10 W/(K*m)  th_cond=0.8 W/(m*K)  th_cond_TLU=[413, 401, 392, 383, 371, 357, 342] W/(K*m)  temp_TLU=[200, 273, 400, 600, 800, 1000, 1200] K  T_specify=off  T_priority=None  T=0 K  T_nominal_specify=off  T_nominal_value=1  T_nominal_unit=K  Q_specify=off  Q_priority=None  Q=0 J/s  Q_nominal_specify=off  Q_nominal_value=1  Q_nominal_unit=J/s
  WiA-WiC Convection : fl_lib/Thermal/Thermal Elements/Convective Heat Transfer  thermal_type=foundation.enum.constant_variable.constant  area=0.004 m^2  heat_tr_coeff=2 W/(m^2 * K)  min_heat_tr_coeff=1e-3 W/(K*m^2)  T_specify=off  T_priority=None  T=0 K  T_nominal_specify=off  T_nominal_value=1  T_nominal_unit=K  Q_specify=off  Q_priority=None  Q=0 J/s  Q_nominal_specify=off  Q_nominal_value=1  Q_nominal_unit=J/s
  WiB-Amb Convection : fl_lib/Thermal/Thermal Elements/Convective Heat Transfer  thermal_type=foundation.enum.constant_variable.constant  area=0.1 m^2  heat_tr_coeff=0.2 W/(m^2 * K)  min_heat_tr_coeff=1e-3 W/(K*m^2)  T_specify=off  T_priority=None  T=0 K  T_nominal_specify=off  T_nominal_value=1  T_nominal_unit=K  Q_specify=off  Q_priority=None  Q=0 J/s  Q_nominal_specify=off  Q_nominal_value=1  Q_nominal_unit=J/s
  WiB-Rot Convection : fl_lib/Thermal/Thermal Elements/Convective Heat Transfer  thermal_type=foundation.enum.constant_variable.constant  area=0.02 m^2  heat_tr_coeff=2 W/(m^2 * K)  min_heat_tr_coeff=1e-3 W/(K*m^2)  T_specify=off  T_priority=None  T=0 K  T_nominal_specify=off  T_nominal_value=1  T_nominal_unit=K  Q_specify=off  Q_priority=None  Q=0 J/s  Q_nominal_specify=off  Q_nominal_value=1  Q_nominal_unit=J/s
  WiB-WiC Conduction : fl_lib/Thermal/Thermal Elements/Conductive Heat Transfer  thermal_type=foundation.enum.ConstantVariableTabulated.Constant  wall_geometry=foundation.enum.ConductionWallGeometry.Planar  area=0.002 m^2  thickness=0.1 m  d_in=0.05 m  d_out=0.1 m  L=1 m  th_cond_min=10 W/(K*m)  th_cond=0.8 W/(m*K)  th_cond_TLU=[413, 401, 392, 383, 371, 357, 342] W/(K*m)  temp_TLU=[200, 273, 400, 600, 800, 1000, 1200] K  T_specify=off  T_priority=None  T=0 K  T_nominal_specify=off  T_nominal_value=1  T_nominal_unit=K  Q_specify=off  Q_priority=None  Q=0 J/s  Q_nominal_specify=off  Q_nominal_value=1  Q_nominal_unit=J/s
  WiB-WiC Convection : fl_lib/Thermal/Thermal Elements/Convective Heat Transfer  thermal_type=foundation.enum.constant_variable.constant  area=0.004 m^2  heat_tr_coeff=2 W/(m^2 * K)  min_heat_tr_coeff=1e-3 W/(K*m^2)  T_specify=off  T_priority=None  T=0 K  T_nominal_specify=off  T_nominal_value=1  T_nominal_unit=K  Q_specify=off  Q_priority=None  Q=0 J/s  Q_nominal_specify=off  Q_nominal_value=1  Q_nominal_unit=J/s
  WiC-Amb Convection : fl_lib/Thermal/Thermal Elements/Convective Heat Transfer  thermal_type=foundation.enum.constant_variable.constant  area=0.1 m^2  heat_tr_coeff=0.2 W/(m^2 * K)  min_heat_tr_coeff=1e-3 W/(K*m^2)  T_specify=off  T_priority=None  T=0 K  T_nominal_specify=off  T_nominal_value=1  T_nominal_unit=K  Q_specify=off  Q_priority=None  Q=0 J/s  Q_nominal_specify=off  Q_nominal_value=1  Q_nominal_unit=J/s
  WiC-Rot Convection : fl_lib/Thermal/Thermal Elements/Convective Heat Transfer  thermal_type=foundation.enum.constant_variable.constant  area=0.02 m^2  heat_tr_coeff=2 W/(m^2 * K)  min_heat_tr_coeff=1e-3 W/(K*m^2)  T_specify=off  T_priority=None  T=0 K  T_nominal_specify=off  T_nominal_value=1  T_nominal_unit=K  Q_specify=off  Q_priority=None  Q=0 J/s  Q_nominal_specify=off  Q_nominal_value=1  Q_nominal_unit=J/s
  Rotor : PMIOPort  Side=Left
  Winding C : PMIOPort  Port=2  Side=Right
  Winding B : PMIOPort  Port=3  Side=Right
  Winding A : PMIOPort  Port=4  Side=Right
  Env : PMIOPort  Port=5  Side=Left
  connections:
  WiA-Rot Convection/RConn1 -- Sensing Temperature WiA/LConn1 -- WiA-WiC Conduction/RConn1 -- WiA-WiC Convection/RConn1 -- WiA-WiB Convection/LConn1 -- WiA-WiB Conduction/LConn1 -- WiA-Amb Convection/LConn1 -- Winding A/RConn1
  Rotor/RConn1 -- Sensing Temperature Rot/LConn1 -- WiC-Rot Convection/LConn1 -- WiB-Rot Convection/LConn1 -- WiA-Rot Convection/LConn1
  WiA-WiB Convection/RConn1 -- WiA-WiB Conduction/RConn1 -- Sensing Temperature WiB/LConn1 -- WiB-Rot Convection/RConn1 -- Winding B/RConn1 -- WiB-Amb Convection/LConn1 -- WiB-WiC Conduction/LConn1 -- WiB-WiC Convection/LConn1
  WiC-Rot Convection/RConn1 -- Winding C/RConn1 -- WiB-WiC Conduction/RConn1 -- WiB-WiC Convection/RConn1 -- WiC-Amb Convection/LConn1 -- WiA-WiC Convection/LConn1 -- WiA-WiC Conduction/LConn1 -- Sensing Temperature WiC/LConn1
  WiA-Amb Convection/RConn1 -- Env/RConn1 -- WiC-Amb Convection/RConn1 -- WiB-Amb Convection/RConn1

== system IntegratedStarterGenerator_lithium_ion/DCDC Buck Converter/Sensor V 12V ==
  PS-Simulink Converter5 : nesl_utility/PS-Simulink Converter  PhysicalDomain=network_engine_domain  SubClassName=ps_output  LeftPortType=input  RightPortType=output  PseudoPeriodic=off  Frequencies=[]  VectorFormat=1-D array  Unit=V  AffineConversion=off
  Voltage Sensor : fl_lib/Electrical/Electrical Sensors/Voltage Sensor
  + : PMIOPort  Side=Left
  - : PMIOPort  Port=2  Side=Right
  vdc : Outport  VectorParamsAs1DForOutWhenUnconnected=off
  wires:
  PS-Simulink Converter5/1 -> vdc/1
  connections:
  +/RConn1 -- Voltage Sensor/LConn1
  PS-Simulink Converter5/LConn1 -- Voltage Sensor/RConn1
  -/RConn1 -- Voltage Sensor/RConn2

== system IntegratedStarterGenerator_lithium_ion/DCDC Controller/PWM Generation ==
  DC : Inport
  Counter Limited : simulink/Sources/Counter Limited  uplimit=1/(f*Ts)  tsamp=Ts
  Data Type Conversion1 : DataTypeConversion  SaturateOnIntegerOverflow=off  RndMeth=Floor
  Data Type Conversion2 : DataTypeConversion  SaturateOnIntegerOverflow=off  RndMeth=Floor
  Gain : Gain  Gain=f*Ts
  Relational Operator : RelationalOperator  OutDataTypeStr=boolean  RndMeth=Simplest  InputSameDT=off
  PWM : Outport  VectorParamsAs1DForOutWhenUnconnected=off
  wires:
  Counter Limited/1 -> Data Type Conversion1/1
  Gain/1 -> Relational Operator/2
  Data Type Conversion2/1 -> PWM/1
  Relational Operator/1 -> Data Type Conversion2/1
  DC/1 -> Relational Operator/1
  Data Type Conversion1/1 -> Gain/1

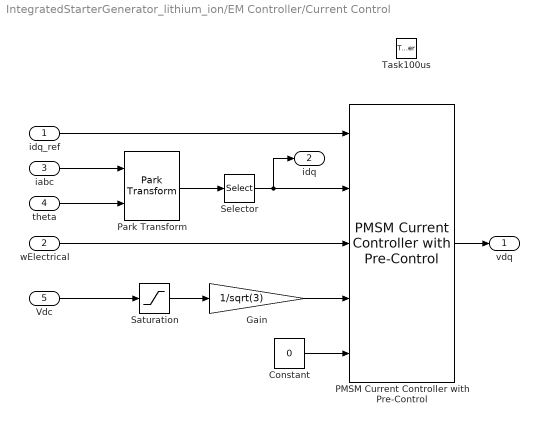
== system IntegratedStarterGenerator_lithium_ion/EM Controller/Current Control ==
  idq_ref : Inport
  wElectrical : Inport  Port=2
  iabc : Inport  Port=3
  theta : Inport  Port=4
  Vdc : Inport  Port=5
  Task100us : TriggerPort  TriggerType=function-call  VariantControl=Variant  PortDimensions=1
  Constant : Constant  Value=0  SampleTime=-1
  Gain : Gain  Gain=1/sqrt(3)
  PMSM Current Controller with Pre-Control : eePmsmCurrentController/PMSM Current Controller with Pre-Control  Kp_id=Kp_id  Ki_id=Ki_id  Kaw_id=1  Kp_iq=Kp_iq  Ki_iq=Ki_iq  Kaw_iq=1  Ts=-1  Tsd=Tsi  AxisPrio=Q-axis  ActZC=on  ActFF=on  idVect=[-40, 0, 40]  iqVect=[-40, 0, 40]  LdMatrix=Ld * ones(3, 3)  LqMatrix=Lq * ones(3, 3)  psimMatrix=psim * ones(3, 3)
  Park Transform : eeTransforms/Park Transform  AxisAlignment=Q-axis  PowerInvariant=off
  Saturation : Saturate  UpperLimit=VDC_VECT(17)  LowerLimit=VDC_VECT(1)  ZeroCross=off
  Selector : Selector  InputPortWidth=3  IndexOptions=Index vector (dialog)  Indices=[1 2]  OutputSizes=1
  vdq : Outport  VectorParamsAs1DForOutWhenUnconnected=off
  idq : Outport  Port=2  VectorParamsAs1DForOutWhenUnconnected=off
  wires:
  iabc/1 -> Park Transform/1
  Saturation/1 -> Gain/1
  Park Transform/1 -> Selector/1
  theta/1 -> Park Transform/2
  Vdc/1 -> Saturation/1
  idq_ref/1 -> PMSM Current Controller with Pre-Control/1
  PMSM Current Controller with Pre-Control/1 -> vdq/1
  wElectrical/1 -> PMSM Current Controller with Pre-Control/3
  Gain/1 -> PMSM Current Controller with Pre-Control/4
  Constant/1 -> PMSM Current Controller with Pre-Control/5
  Selector/1 -> idq/1, PMSM Current Controller with Pre-Control/2

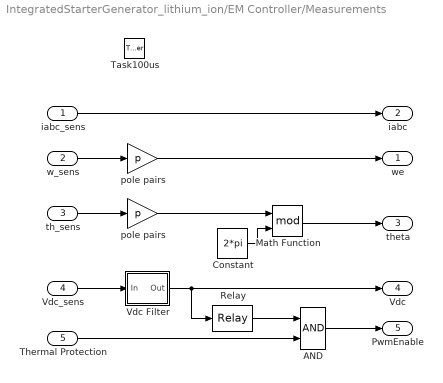
== system IntegratedStarterGenerator_lithium_ion/EM Controller/Measurements ==
  iabc_sens : Inport
  w_sens : Inport  Port=2
  th_sens : Inport  Port=3
  Vdc_sens : Inport  Port=4
  Thermal Protection : Inport  Port=5
  Task100us : TriggerPort  TriggerType=function-call  VariantControl=Variant  PortDimensions=1
  AND : Logic  IconShape=distinctive  AllPortsSameDT=off  OutDataTypeStr=boolean
  Constant : Constant  Value=2*pi  SampleTime=-1
  Math Function : Math  Operator=mod  SignedPower=on
  Relay : Relay  OnSwitchValue=VDC_VECT(1)  OffSwitchValue=0.5*VDC_VECT(1)  ZeroCross=off
  Vdc Filter : Subsystem  mask(Discrete first-order filter (Low-pass)){T=0.005, Ts=1e-4}
      mask prompts: T "Time constant (s):"; Ts "Sample time (s):"
      mask help: This block implements a discrete low-pass filter. To calculate the coefficients, the block discretises a continuous low-pass filter using the Tustin method.
      mask init:
      | num = [ Ts/(2*T + Ts), Ts/(2*T + Ts)];
      | den = [ 1, -(2*T - Ts)/(2*T + Ts)];
  pole pairs : Gain  Gain=p
  "pole pairs " : Gain  Gain=p
  we : Outport  VectorParamsAs1DForOutWhenUnconnected=off
  iabc : Outport  Port=2  VectorParamsAs1DForOutWhenUnconnected=off
  theta : Outport  Port=3  VectorParamsAs1DForOutWhenUnconnected=off
  Vdc : Outport  Port=4  VectorParamsAs1DForOutWhenUnconnected=off
  PwmEnable : Outport  Port=5  VectorParamsAs1DForOutWhenUnconnected=off
  wires:
  w_sens/1 -> pole pairs/1
  iabc_sens/1 -> iabc/1
  pole pairs/1 -> we/1
  Constant/1 -> Math Function/2
  Math Function/1 -> theta/1
  th_sens/1 -> "pole pairs "/1
  "pole pairs "/1 -> Math Function/1
  Vdc_sens/1 -> Vdc Filter/1(In)
  Vdc Filter/1(Out) -> Vdc/1, Relay/1
  Thermal Protection/1 -> AND/2
  Relay/1 -> AND/1
  AND/1 -> PwmEnable/1

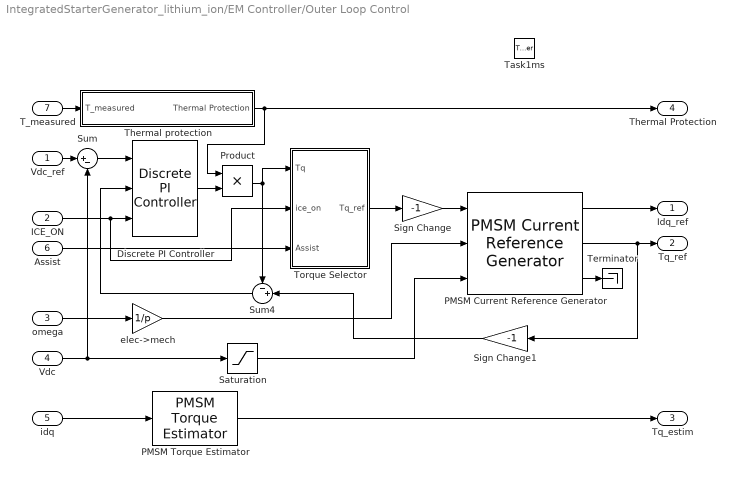
== system IntegratedStarterGenerator_lithium_ion/EM Controller/Outer Loop Control ==
  Vdc_ref : Inport
  ICE_ON : Inport  Port=2
  omega : Inport  Port=3
  Vdc : Inport  Port=4
  idq : Inport  Port=5
  Assist : Inport  Port=6
  T_measured : Inport  Port=7
  Task1ms : TriggerPort  TriggerType=function-call  VariantControl=Variant  PortDimensions=1
  Discrete PI Controller : eeDiscretePi/Discrete PI Controller  Kp=Kp_vdc  Ki=Ki_vdc  Kaw=1  x0=0  Ts=-1
  PMSM Current Reference Generator : eePmsmCurrentReferenceGen/PMSM Current Reference Generator  Vnom=12  Pmax=Pmax  Tmax=Tmax  Ts=-1  RefType=Zero d-axis control  rpmVec=RPM_VECT  TqVec=TQ_VECT  VdcVec=VDC_VECT  PWMMode=SVM: space vector modulation  ModFactor=1  idMatrix=ID_MAP  iqMatrix=IQ_MAP  p=3  psim=psim  Ld=0.00024  Lq=0.00029  Rs=0.01  RefExpEnable=0
  PMSM Torque Estimator : eePmsmTorqueEstimator/PMSM Torque Estimator  ParamType=Constant parameters  p=p  idVect=[-200, 200]  iqVect=[-200, 200]  LdMatrix=0.0002 * ones(2, 2)  LqMatrix=0.0002 * ones(2, 2)  psimMatrix=0.04 * ones(2, 2)  Ld=Ld  Lq=Lq  psim=psim  Ts=-1
  Product : Product
  Saturation : Saturate  UpperLimit=VDC_VECT(17)  LowerLimit=VDC_VECT(1)  LinearizeAsGain=off  ZeroCross=off
  Sign Change : Gain  Gain=-1
  Sign Change1 : Gain  Gain=-1
  Sum : Sum  Inputs=|+-
  Sum4 : Sum  Inputs=-+|
  Terminator : Terminator
  Thermal protection : Subsystem
  Torque Selector : Subsystem
  elec->mech : Gain  Gain=1/p
  Idq_ref : Outport  VectorParamsAs1DForOutWhenUnconnected=off
  Tq_ref : Outport  Port=2  VectorParamsAs1DForOutWhenUnconnected=off
  Tq_estim : Outport  Port=3  VectorParamsAs1DForOutWhenUnconnected=off
  Thermal Protection : Outport  Port=4
  wires:
  Sum/1 -> Discrete PI Controller/1
  Vdc_ref/1 -> Sum/1
  Saturation/1 -> PMSM Current Reference Generator/3
  PMSM Torque Estimator/1 -> Tq_estim/1
  omega/1 -> elec->mech/1
  idq/1 -> PMSM Torque Estimator/1
  Sum4/1 -> Discrete PI Controller/2
  ICE_ON/1 -> Torque Selector/2(ice_on), Discrete PI Controller/3
  Vdc/1 -> Saturation/1, Sum/2
  elec->mech/1 -> PMSM Current Reference Generator/2
  Torque Selector/1(Tq_ref) -> Sign Change/1
  PMSM Current Reference Generator/1 -> Idq_ref/1
  PMSM Current Reference Generator/3 -> Terminator/1
  Sign Change/1 -> PMSM Current Reference Generator/1
  Sign Change1/1 -> Sum4/2
  Assist/1 -> Torque Selector/3(Assist)
  PMSM Current Reference Generator/2 -> Tq_ref/1, Sign Change1/1
  Discrete PI Controller/1 -> Product/2
  Product/1 -> Sum4/1, Torque Selector/1(Tq)
  T_measured/1 -> Thermal protection/1(T_measured)
  Thermal protection/1(Thermal Protection) -> Product/1, Thermal Protection/1

== system IntegratedStarterGenerator_lithium_ion/Scopes/Assist_counter ==
  soc : Inport
  assist_on : Inport  Port=2
  ICE Start [0,1] : Inport  Port=3
  Compare To Constant : simulink/Logic and Bit Operations/Compare To Constant  relop=<  const=0.2  OutDataTypeStr=boolean
  Counter : dspswit3/Counter  Direction=Up  CountEvent=Rising edge  CounterSize=16 bits  MaxCount=255  InitialCount=0  Output=Count  HitValue=32  ResetInput=off  SamplesPerFrame=1  Ts=1  CntDtype=double  HitDtype=Logical
  Memory : Memory  InheritSampleTime=on  LinearizeAsDelay=on
  NOT : Logic  Operator=NOT  IconShape=distinctive  AllPortsSameDT=off  OutDataTypeStr=boolean
  OR : Logic  Operator=OR  IconShape=distinctive  AllPortsSameDT=off  OutDataTypeStr=boolean
  Product2 : Product  Inputs=3
  assist_count : Outport
  wires:
  NOT/1 -> Product2/1
  Product2/1 -> Counter/1
  OR/1 -> Memory/1, NOT/1
  Memory/1 -> OR/1
  Compare To Constant/1 -> OR/2
  soc/1 -> Compare To Constant/1
  ICE Start [0,1]/1 -> Product2/3
  assist_on/1 -> Product2/2
  Counter/1 -> assist_count/1

== system IntegratedStarterGenerator_lithium_ion/Scopes/SOC Calculation ==
  I [A] : Inport
  1/(nominal battery capacity) : Gain  Gain=1/(12*36)
  Abs : Abs  SaturateOnIntegerOverflow=off
  Discrete-Time Integrator : DiscreteIntegrator  IntegratorMethod=Integration: Backward Euler  InitialCondition=0.8  SampleTime=0.0001  LimitOutput=on  UpperSaturationLimit=1  LowerSaturationLimit=0  ICPrevOutput=DiscIntNeverNeededParam  ICPrevScaledInput=DiscIntNeverNeededParam
  Gain : Gain  Gain=1/6
  Gain1 : Gain  Gain=-1
  Gain2 : Gain  Gain=-1
  Math Function : Math  Operator=pow
  Peukert's constant : Constant  Value=1.05  SampleTime=-1
  Sign : Signum
  Switch : Switch  Criteria=u2 > Threshold  SaturateOnIntegerOverflow=off  InputSameDT=off
  SOC [0,1] : Outport  VectorParamsAs1DForOutWhenUnconnected=off
  wires:
  Abs/1 -> Gain/1
  I [A]/1 -> Abs/1, Sign/1, Switch/3
  Gain1/1 -> Switch/2
  Math Function/1 -> Gain2/1
  Sign/1 -> Gain1/1
  Gain2/1 -> Switch/1
  Peukert's constant/1 -> Math Function/2
  Gain/1 -> Math Function/1
  Switch/1 -> 1/(nominal battery capacity)/1
  1/(nominal battery capacity)/1 -> Discrete-Time Integrator/1
  Discrete-Time Integrator/1 -> SOC [0,1]/1

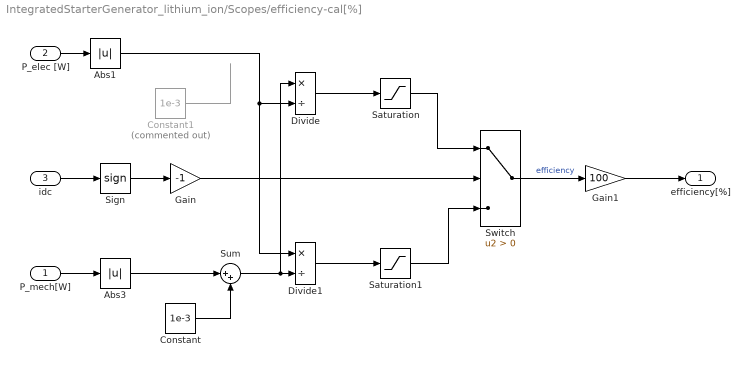
== system IntegratedStarterGenerator_lithium_ion/Scopes/efficiency-cal[%] ==
  P_mech[W] : Inport
  P_elec [W] : Inport  Port=2
  idc : Inport  Port=3
  Abs1 : Abs  ZeroCross=off  SaturateOnIntegerOverflow=off
  Abs3 : Abs  ZeroCross=off  SaturateOnIntegerOverflow=off
  Constant : Constant  Value=1e-3  SampleTime=-1
  Constant1 : Constant  Commented=on  Value=1e-3  SampleTime=-1
  Divide : Product  Inputs=*/
  Divide1 : Product  Inputs=*/
  Gain : Gain  Gain=-1
  Gain1 : Gain  Gain=100
  Saturation : Saturate  UpperLimit=1  LowerLimit=0  LinearizeAsGain=off  ZeroCross=off
  Saturation1 : Saturate  UpperLimit=1  LowerLimit=0  LinearizeAsGain=off  ZeroCross=off
  Sign : Signum
  Sum : Sum  Inputs=|++
  Switch : Switch  Criteria=u2 > Threshold  SaturateOnIntegerOverflow=off  InputSameDT=off
  efficiency[%] : Outport
  wires:
  Divide/1 -> Saturation/1
  Sign/1 -> Gain/1
  Divide1/1 -> Saturation1/1
  Switch/1 -> Gain1/1  "efficiency"
  Constant/1 -> Sum/2
  Constant1/1 -> ?
  Saturation1/1 -> Switch/3
  Saturation/1 -> Switch/1
  Abs3/1 -> Sum/1
  Abs1/1 -> Divide1/1, Divide/2
  idc/1 -> Sign/1
  Gain/1 -> Switch/2
  P_mech[W]/1 -> Abs3/1
  P_elec [W]/1 -> Abs1/1
  Gain1/1 -> efficiency[%]/1
  Sum/1 -> Divide/1, Divide1/2

== system IntegratedStarterGenerator_lithium_ion/Thermal model/Sensing Temperature Rot ==
  PS-Simulink Converter : nesl_utility/PS-Simulink Converter  PhysicalDomain=network_engine_domain  SubClassName=ps_output  LeftPortType=input  RightPortType=output  PseudoPeriodic=off  Frequencies=[]  VectorFormat=1-D array  Unit=degC  AffineConversion=on
  Temperature Sensor : fl_lib/Thermal/Thermal Sensors/Temperature Sensor  temperature_measure=foundation.enum.MeasurementReference.difference
  ThRef : fl_lib/Thermal/Thermal Elements/Thermal Reference
  H : PMIOPort  Side=Left
  tag scope: TR=global
  wires:
  PS-Simulink Converter/1 -> [TR]
  connections:
  Temperature Sensor/RConn2 -- PS-Simulink Converter/LConn1
  ThRef/LConn1 -- Temperature Sensor/RConn1
  H/RConn1 -- Temperature Sensor/LConn1
